simulink library "pwm_deadtime_compensation_lib"  (R2023b)
settings: Solver=VariableStepAuto  StartTime=0.0  StopTime=10.0  RelTol=1e-3
values from neighbouring files (symbols this model uses):
  DeadtimeCompCurrentInvRange_1perA = 12.5    [pwm_deadtime_compensation_interface.sldd]
  DeadtimeCompCurrentZero_A = 0.019999999552965164    [pwm_deadtime_compensation_interface.sldd]
  DeadtimeCompDuty = 0.0099999997764825821    [pwm_deadtime_compensation_interface.sldd]
  DeadtimeCompEnable = 1.0    [pwm_deadtime_compensation_interface.sldd]
  DeadtimeCompPolarity = -1.0    [pwm_deadtime_compensation_interface.sldd]
settings Model: Creator=user  LastModifiedBy=user

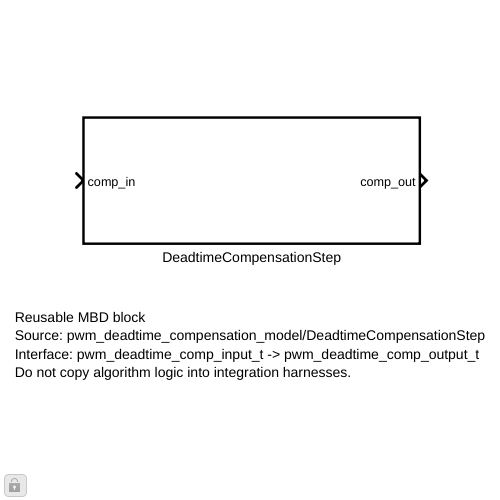
[thumbnail: Simulink's stored preview of the top-level diagram]
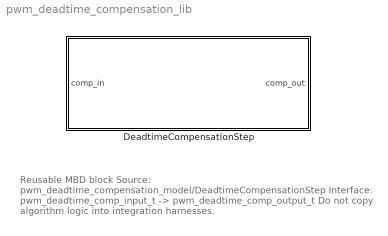
== system pwm_deadtime_compensation_lib ==
  note: Reusable MBD block
      | Source: pwm_deadtime_compensation_model/DeadtimeCompensationStep
      | Interface: pwm_deadtime_comp_input_t -> pwm_deadtime_comp_output_t
      | Do not copy algorithm logic into integration harnesses.
  DeadtimeCompensationStep : Subsystem  TreatAsAtomicUnit=on  RTWFcnName=DeadtimeCompensationStep  RTWFileName=DeadtimeCompensationStep
      settings: RTWFcnNameOpts=User specified  RTWFileNameOpts=User specified

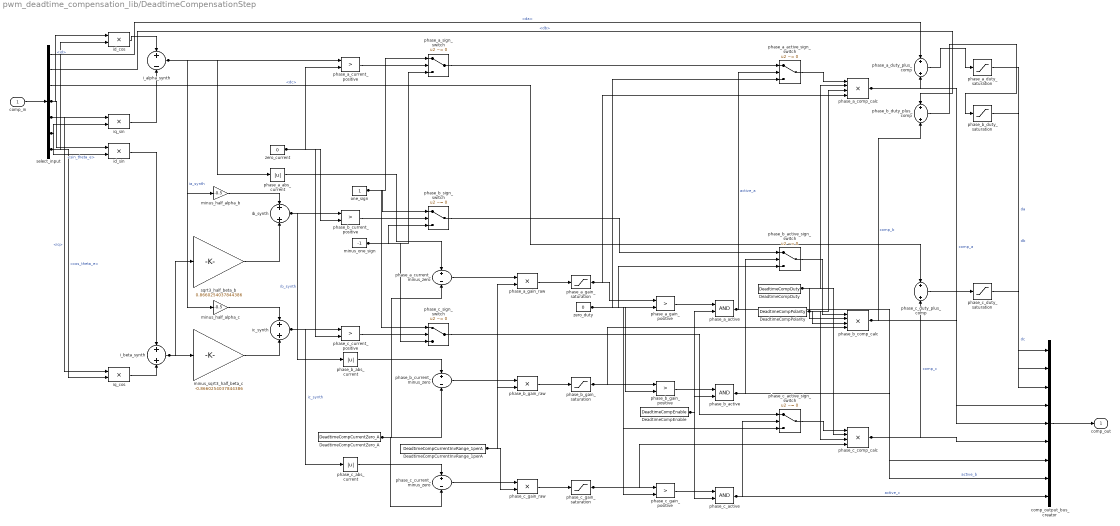
== system pwm_deadtime_compensation_lib/DeadtimeCompensationStep ==
  comp_in : Inport  OutDataTypeStr=Bus: pwm_deadtime_comp_input_t  PortDimensions=1  BusOutputAsStruct=on
  DeadtimeCompCurrentInvRange_1perA : Constant  Value=DeadtimeCompCurrentInvRange_1perA  OutDataTypeStr=T_DeadtimeCompDuty  SampleTime=-1
  DeadtimeCompCurrentZero_A : Constant  Value=DeadtimeCompCurrentZero_A  OutDataTypeStr=T_DeadtimeCompCurrent  SampleTime=-1
  DeadtimeCompDuty : Constant  Value=DeadtimeCompDuty  OutDataTypeStr=T_DeadtimeCompDuty  SampleTime=-1
  DeadtimeCompEnable : Constant  Value=DeadtimeCompEnable  OutDataTypeStr=T_DeadtimeCompBool  SampleTime=-1
  DeadtimeCompPolarity : Constant  Value=DeadtimeCompPolarity  OutDataTypeStr=T_DeadtimeCompDuty  SampleTime=-1
  comp_output_bus_creator : BusCreator  Inputs=9  OutDataTypeStr=Bus: pwm_deadtime_comp_output_t  NonVirtualBus=on
  i_alpha_synth : Sum  Inputs=+-  OutDataTypeStr=T_DeadtimeCompCurrent
  i_beta_synth : Sum  OutDataTypeStr=T_DeadtimeCompCurrent
  ib_synth : Sum  OutDataTypeStr=T_DeadtimeCompCurrent
  ic_synth : Sum  OutDataTypeStr=T_DeadtimeCompCurrent
  id_cos : Product  Inputs=**  OutDataTypeStr=T_DeadtimeCompCurrent
  id_sin : Product  Inputs=**  OutDataTypeStr=T_DeadtimeCompCurrent
  iq_cos : Product  Inputs=**  OutDataTypeStr=T_DeadtimeCompCurrent
  iq_sin : Product  Inputs=**  OutDataTypeStr=T_DeadtimeCompCurrent
  minus_half_alpha_b : Gain  Gain=-0.5  OutDataTypeStr=T_DeadtimeCompCurrent
  minus_half_alpha_c : Gain  Gain=-0.5  OutDataTypeStr=T_DeadtimeCompCurrent
  minus_one_sign : Constant  Value=-1  OutDataTypeStr=T_DeadtimeCompDuty  SampleTime=-1
  minus_sqrt3_half_beta_c : Gain  Gain=-0.8660254037844386  OutDataTypeStr=T_DeadtimeCompCurrent
  one_sign : Constant  OutDataTypeStr=T_DeadtimeCompDuty  SampleTime=-1
  phase_a_abs_current : Abs  SaturateOnIntegerOverflow=off
  phase_a_active : Logic  AllPortsSameDT=off  OutDataTypeStr=T_DeadtimeCompBool
  phase_a_active_sign_switch : Switch  Criteria=u2 ~= 0  OutDataTypeStr=T_DeadtimeCompDuty  SaturateOnIntegerOverflow=off  InputSameDT=off
  phase_a_comp_calc : Product  Inputs=****  OutDataTypeStr=T_DeadtimeCompDuty
  phase_a_current_minus_zero : Sum  Inputs=+-  OutDataTypeStr=T_DeadtimeCompCurrent
  phase_a_current_positive : RelationalOperator  Operator=>  OutDataTypeStr=boolean  RndMeth=Simplest  InputSameDT=off
  phase_a_duty_plus_comp : Sum  OutDataTypeStr=T_DeadtimeCompDuty
  phase_a_duty_saturation : Saturate  UpperLimit=1  LowerLimit=0  OutDataTypeStr=T_DeadtimeCompDuty
  phase_a_gain_positive : RelationalOperator  Operator=>  OutDataTypeStr=boolean  RndMeth=Simplest  InputSameDT=off
  phase_a_gain_raw : Product  Inputs=**  OutDataTypeStr=T_DeadtimeCompDuty
  phase_a_gain_saturation : Saturate  UpperLimit=1  LowerLimit=0  OutDataTypeStr=T_DeadtimeCompDuty
  phase_a_sign_switch : Switch  Criteria=u2 ~= 0  OutDataTypeStr=T_DeadtimeCompDuty  SaturateOnIntegerOverflow=off  InputSameDT=off
  phase_b_abs_current : Abs  SaturateOnIntegerOverflow=off
  phase_b_active : Logic  AllPortsSameDT=off  OutDataTypeStr=T_DeadtimeCompBool
  phase_b_active_sign_switch : Switch  Criteria=u2 ~= 0  OutDataTypeStr=T_DeadtimeCompDuty  SaturateOnIntegerOverflow=off  InputSameDT=off
  phase_b_comp_calc : Product  Inputs=****  OutDataTypeStr=T_DeadtimeCompDuty
  phase_b_current_minus_zero : Sum  Inputs=+-  OutDataTypeStr=T_DeadtimeCompCurrent
  phase_b_current_positive : RelationalOperator  Operator=>  OutDataTypeStr=boolean  RndMeth=Simplest  InputSameDT=off
  phase_b_duty_plus_comp : Sum  OutDataTypeStr=T_DeadtimeCompDuty
  phase_b_duty_saturation : Saturate  UpperLimit=1  LowerLimit=0  OutDataTypeStr=T_DeadtimeCompDuty
  phase_b_gain_positive : RelationalOperator  Operator=>  OutDataTypeStr=boolean  RndMeth=Simplest  InputSameDT=off
  phase_b_gain_raw : Product  Inputs=**  OutDataTypeStr=T_DeadtimeCompDuty
  phase_b_gain_saturation : Saturate  UpperLimit=1  LowerLimit=0  OutDataTypeStr=T_DeadtimeCompDuty
  phase_b_sign_switch : Switch  Criteria=u2 ~= 0  OutDataTypeStr=T_DeadtimeCompDuty  SaturateOnIntegerOverflow=off  InputSameDT=off
  phase_c_abs_current : Abs  SaturateOnIntegerOverflow=off
  phase_c_active : Logic  AllPortsSameDT=off  OutDataTypeStr=T_DeadtimeCompBool
  phase_c_active_sign_switch : Switch  Criteria=u2 ~= 0  OutDataTypeStr=T_DeadtimeCompDuty  SaturateOnIntegerOverflow=off  InputSameDT=off
  phase_c_comp_calc : Product  Inputs=****  OutDataTypeStr=T_DeadtimeCompDuty
  phase_c_current_minus_zero : Sum  Inputs=+-  OutDataTypeStr=T_DeadtimeCompCurrent
  phase_c_current_positive : RelationalOperator  Operator=>  OutDataTypeStr=boolean  RndMeth=Simplest  InputSameDT=off
  phase_c_duty_plus_comp : Sum  OutDataTypeStr=T_DeadtimeCompDuty
  phase_c_duty_saturation : Saturate  UpperLimit=1  LowerLimit=0  OutDataTypeStr=T_DeadtimeCompDuty
  phase_c_gain_positive : RelationalOperator  Operator=>  OutDataTypeStr=boolean  RndMeth=Simplest  InputSameDT=off
  phase_c_gain_raw : Product  Inputs=**  OutDataTypeStr=T_DeadtimeCompDuty
  phase_c_gain_saturation : Saturate  UpperLimit=1  LowerLimit=0  OutDataTypeStr=T_DeadtimeCompDuty
  phase_c_sign_switch : Switch  Criteria=u2 ~= 0  OutDataTypeStr=T_DeadtimeCompDuty  SaturateOnIntegerOverflow=off  InputSameDT=off
  select_input : BusSelector  OutputSignals=da,db,dc,id,iq,sin_theta_e,cos_theta_e
  sqrt3_half_beta_b : Gain  Gain=0.8660254037844386  OutDataTypeStr=T_DeadtimeCompCurrent
  zero_current : Constant  Value=0  OutDataTypeStr=T_DeadtimeCompCurrent  SampleTime=-1
  zero_duty : Constant  Value=0  OutDataTypeStr=T_DeadtimeCompDuty  SampleTime=-1
  comp_out : Outport  OutDataTypeStr=Bus: pwm_deadtime_comp_output_t  PortDimensions=1
  wires:
  phase_b_comp_calc/1 -> comp_output_bus_creator/5, phase_b_duty_plus_comp/2  "comp_b"
  phase_b_active_sign_switch/1 -> phase_b_comp_calc/1
  phase_a_gain_positive/1 -> phase_a_active/1
  phase_b_gain_saturation/1 -> phase_b_comp_calc/4, phase_b_gain_positive/1
  phase_c_gain_positive/1 -> phase_c_active/1
  minus_sqrt3_half_beta_c/1 -> ic_synth/2
  zero_duty/1 -> phase_b_active_sign_switch/3, phase_c_gain_positive/2, phase_c_active_sign_switch/3, phase_a_active_sign_switch/3, phase_a_gain_positive/2, phase_b_gain_positive/2
  phase_c_gain_raw/1 -> phase_c_gain_saturation/1
  phase_a_gain_saturation/1 -> phase_a_comp_calc/4, phase_a_gain_positive/1
  phase_b_gain_raw/1 -> phase_b_gain_saturation/1
  phase_a_gain_raw/1 -> phase_a_gain_saturation/1
  select_input/1 -> phase_a_duty_plus_comp/1  "<da>"
  phase_c_current_minus_zero/1 -> phase_c_gain_raw/1
  phase_c_duty_plus_comp/1 -> phase_c_duty_saturation/1
  DeadtimeCompCurrentInvRange_1perA/1 -> phase_a_gain_raw/2, phase_c_gain_raw/2, phase_b_gain_raw/2
  minus_half_alpha_b/1 -> ib_synth/1
  phase_a_active_sign_switch/1 -> phase_a_comp_calc/1
  phase_b_sign_switch/1 -> phase_b_active_sign_switch/1
  phase_c_comp_calc/1 -> comp_output_bus_creator/6, phase_c_duty_plus_comp/2  "comp_c"
  phase_a_sign_switch/1 -> phase_a_active_sign_switch/1
  phase_c_abs_current/1 -> phase_c_current_minus_zero/1
  phase_c_sign_switch/1 -> phase_c_active_sign_switch/1
  id_sin/1 -> i_beta_synth/1
  id_cos/1 -> i_alpha_synth/1
  select_input/7 -> id_cos/2, iq_cos/2  "<cos_theta_e>"
  zero_current/1 -> phase_a_current_positive/2, phase_c_current_positive/2, phase_b_current_positive/2
  phase_b_current_minus_zero/1 -> phase_b_gain_raw/1
  select_input/6 -> iq_sin/2, id_sin/2  "<sin_theta_e>"
  phase_c_active_sign_switch/1 -> phase_c_comp_calc/1
  comp_in/1 -> select_input/1
  DeadtimeCompPolarity/1 -> phase_c_comp_calc/3, phase_a_comp_calc/3, phase_b_comp_calc/3
  select_input/4 -> id_cos/1, id_sin/1  "<id>"
  i_alpha_synth/1 -> phase_a_current_positive/1, minus_half_alpha_b/1, phase_a_abs_current/1, minus_half_alpha_c/1  "ia_synth"
  phase_a_active/1 -> comp_output_bus_creator/7, phase_a_active_sign_switch/2  "active_a"
  phase_a_comp_calc/1 -> comp_output_bus_creator/4, phase_a_duty_plus_comp/2  "comp_a"
  phase_c_active/1 -> comp_output_bus_creator/9, phase_c_active_sign_switch/2  "active_c"
  phase_b_active/1 -> comp_output_bus_creator/8, phase_b_active_sign_switch/2  "active_b"
  iq_cos/1 -> i_beta_synth/2
  DeadtimeCompEnable/1 -> phase_a_active/2, phase_c_active/2, phase_b_active/2
  phase_b_abs_current/1 -> phase_b_current_minus_zero/1
  select_input/3 -> phase_c_duty_plus_comp/1  "<dc>"
  DeadtimeCompDuty/1 -> phase_a_comp_calc/2, phase_c_comp_calc/2, phase_b_comp_calc/2
  iq_sin/1 -> i_alpha_synth/2
  i_beta_synth/1 -> sqrt3_half_beta_b/1, minus_sqrt3_half_beta_c/1
  phase_c_gain_saturation/1 -> phase_c_comp_calc/4, phase_c_gain_positive/1
  phase_a_abs_current/1 -> phase_a_current_minus_zero/1
  ic_synth/1 -> phase_c_abs_current/1, phase_c_current_positive/1  "ic_synth"
  select_input/5 -> iq_sin/1, iq_cos/1  "<iq>"
  phase_c_duty_saturation/1 -> comp_output_bus_creator/3  "dc"
  minus_one_sign/1 -> phase_a_sign_switch/3, phase_c_sign_switch/3, phase_b_sign_switch/3
  phase_b_gain_positive/1 -> phase_b_active/1
  phase_a_current_minus_zero/1 -> phase_a_gain_raw/1
  one_sign/1 -> phase_c_sign_switch/1, phase_a_sign_switch/1, phase_b_sign_switch/1
  sqrt3_half_beta_b/1 -> ib_synth/2
  minus_half_alpha_c/1 -> ic_synth/1
  select_input/2 -> phase_b_duty_plus_comp/1  "<db>"
  phase_b_current_positive/1 -> phase_b_sign_switch/2
  phase_c_current_positive/1 -> phase_c_sign_switch/2
  phase_a_current_positive/1 -> phase_a_sign_switch/2
  ib_synth/1 -> phase_b_abs_current/1, phase_b_current_positive/1  "ib_synth"
  DeadtimeCompCurrentZero_A/1 -> phase_c_current_minus_zero/2, phase_b_current_minus_zero/2, phase_a_current_minus_zero/2
  phase_a_duty_plus_comp/1 -> phase_a_duty_saturation/1
  phase_b_duty_plus_comp/1 -> phase_b_duty_saturation/1
  phase_a_duty_saturation/1 -> comp_output_bus_creator/1  "da"
  phase_b_duty_saturation/1 -> comp_output_bus_creator/2  "db"
  comp_output_bus_creator/1 -> comp_out/1
